simulink model "realtime"  (R2021a)
settings: Solver=FixedStepDiscrete  StartTime=0.0  StopTime=inf  RelTol=1e-3
libraries: audiosources x1, dspsnks4 x1, dspstat3 x1, deeplib x1, dspsigops x1
settings Model: Creator=Kazuki Matsumoto  LastModifiedBy=Kazuki Matsumoto
settings SolverCC: AlgebraicLoopSolver=TrustRegion  AutoInsertRateTranBlk=on
settings DataIOCC: LimitDataPoints=on  SaveOutput=off  SignalLogging=off  SaveTime=off
settings OptimizationCC: LifeSpan=inf
settings DebuggingCC: AlgebraicLoopMsg=error  SingleTaskRateTransMsg=error  AllowSymbolicDim=off  SFUnexpectedBacktrackingDiag=warning  SFNoUnconditionalDefaultTransitionDiag=warning  SFExecutionAtInitializationDiag=none  SFMachineParentedDataDiag=warning  ArithmeticOperatorsInVariantConditions=warning
settings SFSimCC: SimUseLocalCustomCode=off  CustomCodeUndefinedFunction=UseInterfaceOnly
settings RTWCC: RTWUseLocalCustomCode=off
settings CodeAppCC: StateflowObjectComments=on
settings GRTTargetCC: TargetLangStandard=C89/C90 (ANSI)
settings ConfigComp: CovMetricSettings=dw  CovSaveCumulativeToWorkspaceVar=on  CovSaveSingleToWorkspaceVar=on  CovExternalEMLEnable=off  CovSFcnEnable=off

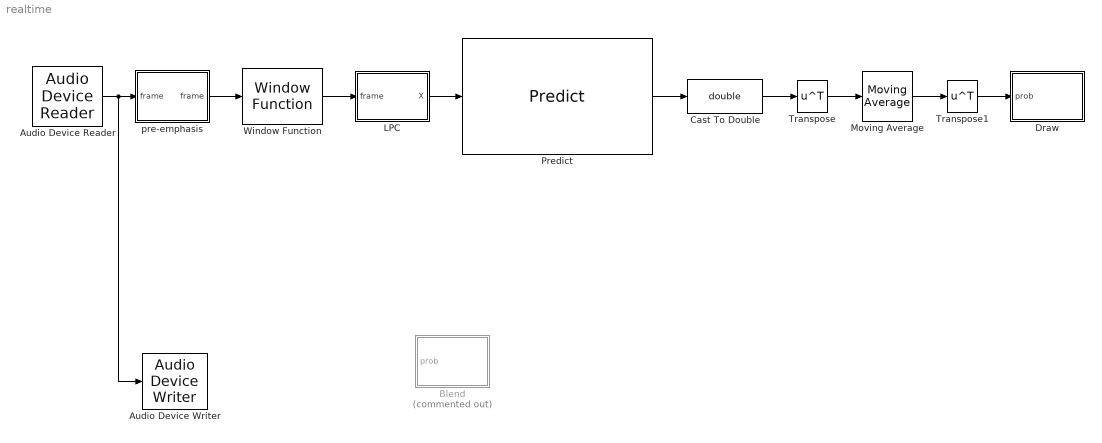
== system realtime ==
  Audio Device Reader : audiosources/Audio Device Reader  Driver=DirectSound  Device=Default  SampleRate=44100  NumChannels=1  SamplesPerFrame=1024  BitDepth=16-bit integer  NumBuffers=10  DefaultInputChannelMapping=on  InputChannelMapping=1:2  OutputNumOverrunSamples=off  OutputDataType=double  DriverIdx=1  DeviceWarnFlag=''
      settings: SourceProductBaseCode=AU
  Audio Device Writer : dspsnks4/Audio Device Writer  Driver=DirectSound  Device=Default  InheritSampleRate=on  SampleRate=44100  BitDepth=16-bit integer  BufferSize=4096  NumBuffers=10  DefaultOutputChannelMapping=on  OutputChannelMapping=1:2  OutputNumUnderrunSamples=off  DriverIdx=1  DeviceWarnFlag=''
  Blend : MATLAB Function  Commented=on  TreatAsAtomicUnit=on
  Cast To Double : DataTypeConversion  OutDataTypeStr=double
  Draw : MATLAB Function  TreatAsAtomicUnit=on
  LPC : MATLAB Function  TreatAsAtomicUnit=on
  Moving Average : dspstat3/Moving Average  Method=Sliding window  ForgettingFactorPort=off  SpecifyWindowLength=on  WindowLength=2  ForgettingFactor=0.9  SimulateUsing=Code generation
  Predict : deeplib/Predict  Network=Network from MAT-file  NetworkFunction=squeezenet  NetworkFilePath=net\net.mat  MiniBatchSize=1  InputDataFormats={ '', '' }  Predictions=on  Activations={}  ForceInterpretedSim=off  EnableDLNetwork=off
      settings: SourceProductBaseCode=NN
  Transpose : Math  Operator=transpose  SaturateOnIntegerOverflow=on
  Transpose1 : Math  Operator=transpose  SaturateOnIntegerOverflow=on
  Window Function : dspsigops/Window Function  winmode=Apply window to input  wintype=Hamming  sampmode=Continuous  samptime=1  N=64  Rs=50  beta=10  winsamp=Symmetric  UserWindow=hamming  OptParams=off  UserParams={'symmetric'}  dataType=double  isSigned=on  wordLen=16  udDataType=sfix(16)  fracBitsMode=Best precision  numFracBits=15  roundingMode=Floor  overflowMode=off  numSidelobes=4  sidelobeLevel=-30
      settings: SourceProductBaseCode=DS
  pre-emphasis : MATLAB Function  TreatAsAtomicUnit=on
  wires:
  LPC/1(X) -> Predict/1
  Audio Device Reader/1 -> Audio Device Writer/1, pre-emphasis/1("frame ")
  pre-emphasis/1(frame) -> Window Function/1
  Window Function/1 -> LPC/1(frame)
  Predict/1 -> Cast To Double/1
  Cast To Double/1 -> Transpose/1
  Transpose/1 -> Moving Average/1
  Moving Average/1 -> Transpose1/1
  Transpose1/1 -> Draw/1(prob)

== matlab function realtime/LPC ==
  data: frame input; X output
function X = fcn(frame)
    %lpcを外部関数とする
    coder.extrinsic("lpc");
    
    %LPC係数の計算
    %外部関数から得た数値にはいろいろと制約があるっぽかった
    %（例えば配列のスライスが使えなかった）ので，あらかじめ作成した変数に
    %代入することでこれを回避してます (何かいい方法があればぜひ教えてください！）
    N = 128;
    A = zeros(N+1,1);
    A = lpc(frame,N);
    X = A(2:end);

== matlab function realtime/pre-emphasis ==
  data: frame input; frame output
function frame = fcn(frame)
    %プリエンファシス
    preemph = [1 -0.97];
    frame = filter(preemph,1,frame);

== matlab function realtime/Blend ==
  data: prob input
function fnc(prob)
    vowels = ['a', 'i', 'u', 'e', 'o', 'n', '-'];
    coeff = 0.3;
    
    persistent point
    if isempty(point)
        point = [[0; 3] [0; 1] [1; 2] [0; 2] [1; 3] [0; 0] [0; 0]];
    end
    persistent pos
    if isempty(pos)
        pos = [0; 0];
    end
    
    target = point*prob;
    pos = pos*(1-coeff)+target*coeff;
    
    plot(pos(1),pos(2),"marker",".","markersize",16);
    hold on
    for i = 1:length(vowels)-1
        text(point(1,i),point(2,i),vowels(i),'FontSize',floor(prob(i)*20+10));
    end
    xlim([-1,2]);
    ylim([-0.5,3.5])
    hold off
    drawnow
    
    position = pos;
    
end

== matlab function realtime/Draw ==
  data: prob input
function fcn(prob)
    size = 500;

    %コード生成に対応しない関数を外部関数とする
    coder.extrinsic("append","image");

    %永続関数imgsに画像を格納
    persistent imgs
    if isempty(imgs)
        %音の種類
        vowels = ['a', 'i', 'u', 'e', 'o', 'n', '-'];

        %セル配列imgsを作成
        imgs = cell(length(vowels),1);

        %音の種類ごとに画像を読み込み
        for i = 1:length(vowels)
            %画像を格納する配列を作成
            %注：画像のサイズと合わせる．チャンネル数は基本的に3
            img = uint8(zeros(size,size,3));

            %画像の読み込みと保存
            img = imresize(imread(append('images\',vowels(i),".jpg")),[size,size]);
            imgs{i} = img;
        end
    end

    %値の最も大きい要素のインデックスを取得
    [~,index] = max(prob);

    %取得したインデックスと対応する画像を描画
    image(imgs{index})
    drawnow
